simulink model "a"  (R2016a)
settings: Solver=VariableStepAuto  StartTime=0.0  StopTime=10  RelTol=1e-3
libraries: powerlib_meascontrol x1, powerlib x1
settings Model: Creator=Lenovo  LastModifiedBy=Lenovo

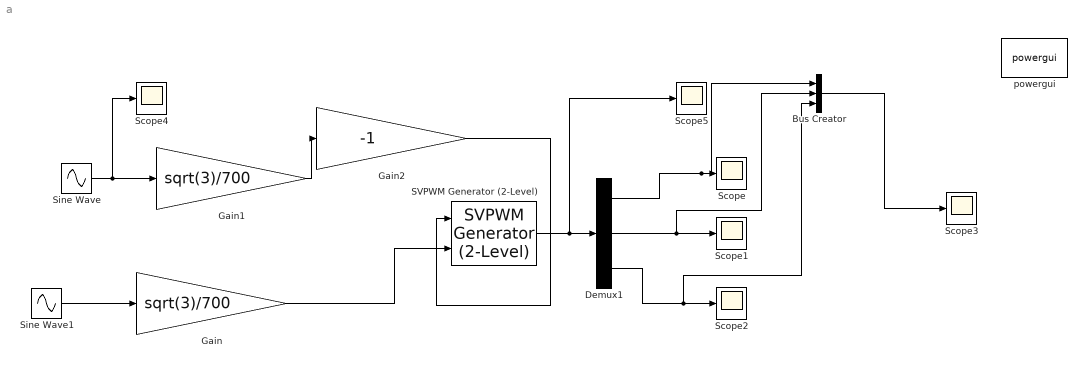
== system a ==
  Bus Creator : BusCreator  Inputs=3
  Demux1 : Demux  Outputs=3
  Gain : Gain  Gain=sqrt(3)/700
  Gain1 : Gain  Gain=sqrt(3)/700
  Gain2 : Gain  Gain=-1
  SVPWM Generator (2-Level) : powerlib_meascontrol/Pulse & Signal Generators/SVPWM Generator (2-Level)  InputType=alpha-beta components  SwitchingPattern=Pattern #1  Fc=50  ParUref=[0.8 -30 50]  Ts=0
  Scope{,1..5} (6 alike) : Scope
  Sine Wave : Sin  Frequency=50  SampleTime=0
  Sine Wave1 : Sin  Amplitude=10  Frequency=50  SampleTime=0
  powergui : powerlib/powergui  Priority=1  SimulationMode=Continuous  SolverType=Tustin/Backward Euler (TBE)  SampleTime=50e-6  frequency=60  SPID=off  DisableSnubberDevices=off  DisableRonSwitches=off  DisableVfSwitches=off  SwTol=0  DisplayEquations=off  Interpol=off  ExternalGateDelay=off  methode=off  Ts=10  FunctionMessages=off  echomessages=off  HookPort=off  EnableUseOfTLC=off  x0status=blocks  frequencyindice=60  Pbase=100e6  ErrMax=1e-4  Iterations=50  UnitsV=kV  UnitsW=MW  buscounter=0  RestoreLinks=warning  ResistiveCurrentMeasurement=off  Frange=[0:2:500]  Ylog=off  Xlog=on  ShowGrid=off  save=off  variable=ZData  structure=0  ZoomFFT=off  StartTime=0.0  cycles=1  DisplayStyle=1  fundamental=60  FreqAxis=off  MaxFrequency=1000  frequencyindicesteady=1  RmsSteady=1  display=off
  wires:
  SVPWM Generator (2-Level)/1 -> Scope5/1, Demux1/1
  Sine Wave1/1 -> Gain/1
  Gain/1 -> SVPWM Generator (2-Level)/2
  Sine Wave/1 -> Scope4/1, Gain1/1
  Gain1/1 -> Gain2/1
  Gain2/1 -> SVPWM Generator (2-Level)/1
  Demux1/1 -> Bus Creator/1, Scope/1
  Demux1/2 -> Bus Creator/2, Scope1/1
  Demux1/3 -> Bus Creator/3, Scope2/1
  Bus Creator/1 -> Scope3/1
